simulink model "Kalman_Modular2_Simple"  (R2019b)
settings: Solver=VariableStepAuto  StartTime=0.0  StopTime=combined_model.sim_dur  FixedStep=model.Ts  RelTol=1e-6
undefined symbols (not defined in the file or in its folder): combined_model, model1, model2
libraries: dspsrcs4 x3
settings Model: Creator=isidoraradenkovic  LastModifiedBy=isidoraradenkovic

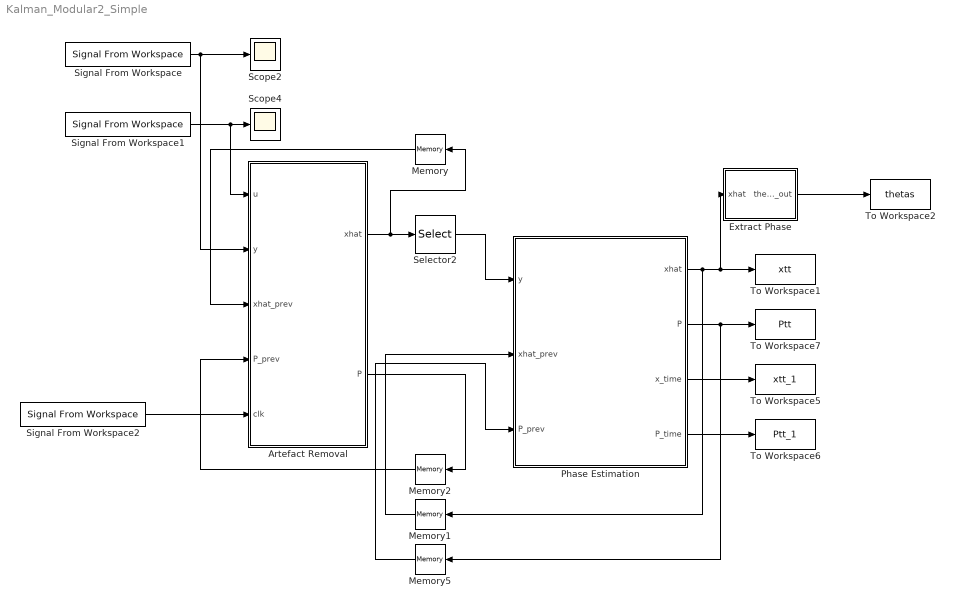
== system Kalman_Modular2_Simple ==
  Artefact Removal : MATLAB Function  TreatAsAtomicUnit=on
  Extract Phase : MATLAB Function  TreatAsAtomicUnit=on
  Memory : Memory  InitialCondition=model1.x_0  InheritSampleTime=on
  Memory1 : Memory  InitialCondition=model2.x_0  InheritSampleTime=on
  Memory2 : Memory  InitialCondition=model1.P0  InheritSampleTime=on
  Memory5 : Memory  InitialCondition=model2.P0  InheritSampleTime=on
  Phase Estimation : MATLAB Function  TreatAsAtomicUnit=on
  Scope2 : Scope
  Scope4 : Scope
  Selector2 : Selector  InputPortWidth=6  IndexOptions=Index vector (dialog)  Indices=[1]  OutputSizes=1
  Signal From Workspace : dspsrcs4/Signal From Workspace  X=input_data  Ts=combined_model.Ts  nsamps=1  OutputAfterFinalValue=Cyclic repetition  ignoreOrWarnInputAndFrameLengths=off  OutputFrames=off
  Signal From Workspace1 : dspsrcs4/Signal From Workspace  X=tms_pulses  Ts=combined_model.Ts  nsamps=1  OutputAfterFinalValue=Cyclic repetition  ignoreOrWarnInputAndFrameLengths=off  OutputFrames=off
  Signal From Workspace2 : dspsrcs4/Signal From Workspace  X=combined_model.clk  Ts=combined_model.Ts  nsamps=1  OutputAfterFinalValue=Cyclic repetition  ignoreOrWarnInputAndFrameLengths=off  OutputFrames=off
  To Workspace1 : ToWorkspace  VariableName=xtt  SampleTime=combined_model.Ts
      settings: Save2DSignal=2-D array (concatenate along first dimension)
  To Workspace2 : ToWorkspace  VariableName=thetas  SampleTime=combined_model.Ts
      settings: Save2DSignal=2-D array (concatenate along first dimension)
  To Workspace5 : ToWorkspace  VariableName=xtt_1  SampleTime=combined_model.Ts
      settings: Save2DSignal=2-D array (concatenate along first dimension)
  To Workspace6 : ToWorkspace  VariableName=Ptt_1  SampleTime=combined_model.Ts
      settings: Save2DSignal=2-D array (concatenate along first dimension)
  To Workspace7 : ToWorkspace  VariableName=Ptt  SampleTime=combined_model.Ts
      settings: Save2DSignal=2-D array (concatenate along first dimension)
  wires:
  Signal From Workspace1/1 -> Artefact Removal/1(u), Scope4/1
  Signal From Workspace/1 -> Artefact Removal/2(y), Scope2/1
  Phase Estimation/2(P) -> To Workspace7/1, Memory5/1
  Artefact Removal/1(xhat) -> Memory/1, Selector2/1
  Extract Phase/1(thetas_out) -> To Workspace2/1
  Memory2/1 -> Artefact Removal/4(P_prev)
  Phase Estimation/4(P_time) -> To Workspace6/1
  Memory1/1 -> Phase Estimation/2(xhat_prev)
  Memory5/1 -> Phase Estimation/3(P_prev)
  Memory/1 -> Artefact Removal/3(xhat_prev)
  Phase Estimation/1(xhat) -> Extract Phase/1(xhat), To Workspace1/1, Memory1/1
  Artefact Removal/2(P) -> Memory2/1
  Selector2/1 -> Phase Estimation/1(y)
  Phase Estimation/3(x_time) -> To Workspace5/1
  Signal From Workspace2/1 -> Artefact Removal/5(clk)

== matlab function Kalman_Modular2_Simple/Phase Estimation ==
  data: xhat output; y input; xhat_prev input; P_prev input; P output; x_time output; P_time output; model2 parameter
function [xhat, P, x_time, P_time] = phase_kalman(y, xhat_prev, P_prev, model2)
x_time = model2.A*xhat_prev;
P_time = model2.A*P_prev*model2.A'+ model2.Q;

K = P_time*(model2.C')*pinv(model2.C*P_time*model2.C' + model2.R);
epsilon = y - model2.C*x_time;

xhat = x_time + K*epsilon;
P = P_time - K*model2.C*P_time;
end

== matlab function Kalman_Modular2_Simple/Extract Phase ==
  settings: sampleTime=combined_model.Ts
  data: xhat input; thetas_out output
function thetas_out  = extract_phase(xhat)

thetas_out = atan2(xhat(2), xhat(1))

== matlab function Kalman_Modular2_Simple/Artefact Removal ==
  data: u input; xhat output; y input; xhat_prev input; P_prev input; clk input size=1; P output; model1 parameter
function [xhat, P] = artefact_kalman(u, y, xhat_prev, P_prev, clk, model1)
Q = model1.Q(((clk-1)*4+1):(clk*4), 1:4)
R = model1.R(clk);

x_time = model1.A*xhat_prev + model1.B*u;
P_time = model1.A*P_prev*model1.A'+ model1.G*Q*model1.G';

K = P_time*(model1.C')*pinv(model1.C*P_time*model1.C' + R);
epsilon = y - model1.C*x_time;

xhat = x_time + K*epsilon;
P = P_time - K*model1.C*P_time;
